simulink model "L06_02"  (R2016a)
settings: Solver=VariableStepAuto  StartTime=0.0  StopTime=10.0  RelTol=1e-3
settings Model: Creator=Student  LastModifiedBy=Student

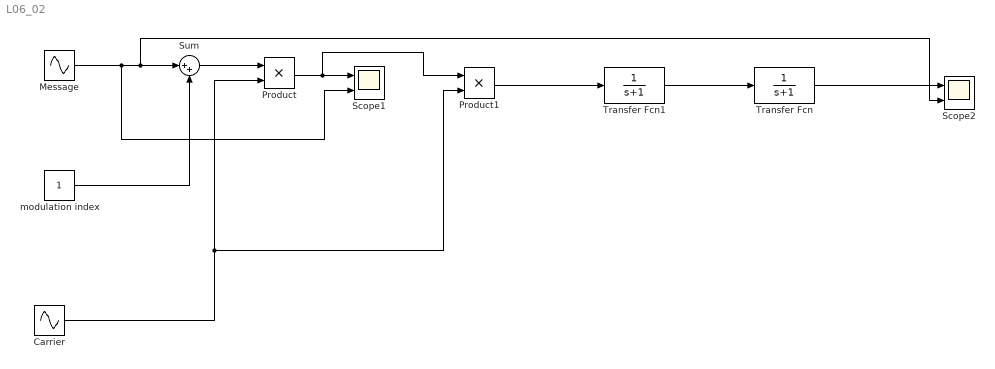
== system L06_02 ==
  Carrier : Sin  Frequency=2  SampleTime=1/5000
  Message : Sin  Frequency=30  Samples=25  SampleTime=1/5000
  Product : Product
  Product1 : Product
  Scope1 : Scope  NumInputPorts=2
  Scope2 : Scope  NumInputPorts=2
  Sum : Sum  Inputs=|++
  Transfer Fcn : TransferFcn  Denominator=[1 1]
  Transfer Fcn1 : TransferFcn  Denominator=[1 1]
  modulation index : Constant
  wires:
  modulation index/1 -> Sum/2
  Message/1 -> Scope1/2, Scope2/2, Sum/1
  Sum/1 -> Product/1
  Carrier/1 -> Product1/2, Product/2
  Product/1 -> Product1/1, Scope1/1
  Product1/1 -> Transfer Fcn1/1
  Transfer Fcn1/1 -> Transfer Fcn/1
  Transfer Fcn/1 -> Scope2/1
